simulink model "Schemabloc"  (R2021a)
settings: Solver=VariableStepAuto  StartTime=0.0  StopTime=10.0  RelTol=1e-3
values from neighbouring files (symbols this model uses):
  BL = 1    [Problematique_APP3S5.m]
  Bm = 0.01    [Problematique_APP3S5.m]
  JL = 1    [Problematique_APP3S5.m]
  Jm = 0.02    [Problematique_APP3S5.m]
  K = 100    [Problematique_APP3S5.m]
  Kb = 0.5    [Problematique_APP3S5.m]
  Ki = 0.5    [Problematique_APP3S5.m]
  La = 0.008    [Problematique_APP3S5.m]
  N = 0.1    [Problematique_APP3S5.m]
  Ra = 8    [Problematique_APP3S5.m]
  tau = 0.01    [Problematique_APP3S5.m]
settings Model: Creator=antho  LastModifiedBy=antho

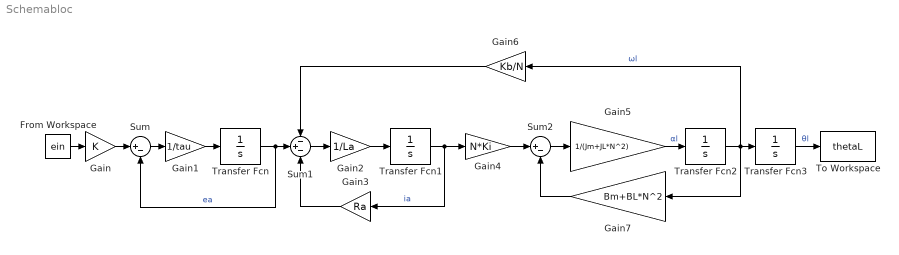
== system Schemabloc ==
  From Workspace : FromWorkspace  VariableName=ein
  Gain : Gain  Gain=K
  Gain1 : Gain  Gain=1/tau
  Gain2 : Gain  Gain=1/La
  Gain3 : Gain  Gain=Ra
  Gain4 : Gain  Gain=N*Ki
  Gain5 : Gain  Gain=1/(Jm+JL*N^2)
  Gain6 : Gain  Gain=Kb/N
  Gain7 : Gain  Gain=Bm+BL*N^2
  Sum : Sum  Inputs=|+-
  Sum1 : Sum  Inputs=-+-
  Sum2 : Sum  Inputs=|+-
  To Workspace : ToWorkspace  VariableName=thetaL  SaveFormat=Timeseries  SampleTime=-1
  Transfer Fcn{,1..3} (4 alike) : TransferFcn  Denominator=[1 0]
  wires:
  Gain/1 -> Sum/1
  From Workspace/1 -> Gain/1
  Sum/1 -> Gain1/1
  Gain1/1 -> Transfer Fcn/1
  Transfer Fcn/1 -> Sum1/2, Sum/2  "ea"
  Sum1/1 -> Gain2/1
  Gain2/1 -> Transfer Fcn1/1
  Gain3/1 -> Sum1/3
  Transfer Fcn1/1 -> Gain4/1, Gain3/1  "ia"
  Gain4/1 -> Sum2/1
  Sum2/1 -> Gain5/1
  Gain5/1 -> Transfer Fcn2/1  "αl"
  Transfer Fcn2/1 -> Transfer Fcn3/1, Gain7/1, Gain6/1  "ωl"
  Transfer Fcn3/1 -> To Workspace/1  "θl"
  Gain6/1 -> Sum1/1
  Gain7/1 -> Sum2/2
